simulink model "Simulation_balance_TEST"  (R2024a)
settings: Solver=ode4  StartTime=0.0  StopTime=5  FixedStep=1/750000  RelTol=1e-3
InitFcn:
  | Initialisation_simulation
values from neighbouring files (symbols this model uses):
  denom_com = [R^2*C^2 3*R*C 1]    [Initialisation_simulation.m]
  denom_cou = [1/(2*pi*165) 1]    [Initialisation_simulation.m]
  denom_pos = [1/(2*pi*80) 1]    [Initialisation_simulation.m]
  gain_com = 0.88    [Initialisation_simulation.m]
  gain_cou = 0.716    [Initialisation_simulation.m]
  gain_mod_cou = Gain_Ampli_Puissance(1)    [Initialisation_simulation.m]
  gain_pos = 1.4925    [Initialisation_simulation.m]
  gain_puis = Gain_Ampli_Puissance(1)    [Initialisation_simulation.m]
  num_com = 1    [Initialisation_simulation.m]
  num_cou = 1    [Initialisation_simulation.m]
  num_pos = 1    [Initialisation_simulation.m]
  offset_com = -2.5    [Initialisation_simulation.m]
  offset_cou = 3.44    [Initialisation_simulation.m]
  offset_pos = -1.6    [Initialisation_simulation.m]
  per_adc = 1/freq_adc    (= 0.000166666666667)    [Initialisation_simulation.m]
  per_pwm = 1/freq_pwm    (= 6.4e-05)    [Initialisation_simulation.m]
  sat_com_max = 5    [Initialisation_simulation.m]
  sat_com_min = -5    [Initialisation_simulation.m]
  sat_cou_max = 5    [Initialisation_simulation.m]
  sat_cou_min = 0    [Initialisation_simulation.m]
  sat_pos_max = 5    [Initialisation_simulation.m]
  sat_pos_min = 0    [Initialisation_simulation.m]
  sat_proc_max = 14e-3    (= 0.014)    [Initialisation_simulation.m]    (also in lookup_table_statespace.m = 1)
  sat_proc_min = 0    [Initialisation_simulation.m]    (also in lookup_table_statespace.m = -1)
  sat_puis_max = 5    [Initialisation_simulation.m]
  sat_puis_min = -5    [Initialisation_simulation.m]
  tension_selon_distance = polyfit(Distance(1:point_final), Tension(1:point_final), 3)    [Initialisation_simulation.m]
undefined symbols (not defined in the file or in its folder): denom_pid_cou, denom_pid_pos, denom_proc, num_pid_cou, num_pid_pos, num_proc
libraries: simulink_extras x2, simulink x1
settings Model: DataTypeOverride=Double  MinMaxOverflowLogging=ForceOff  Creator=johen30  LastModifiedBy=johen30

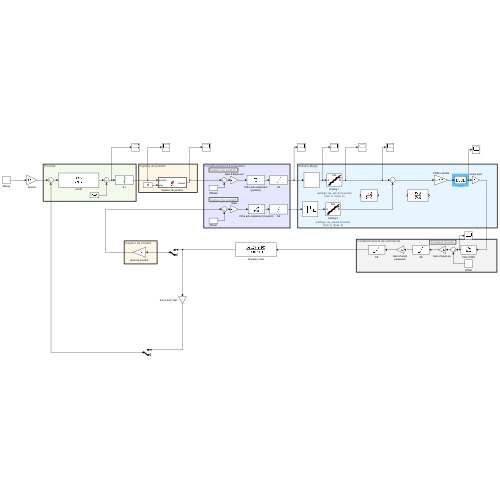
[thumbnail: Simulink's stored preview of the top-level diagram]
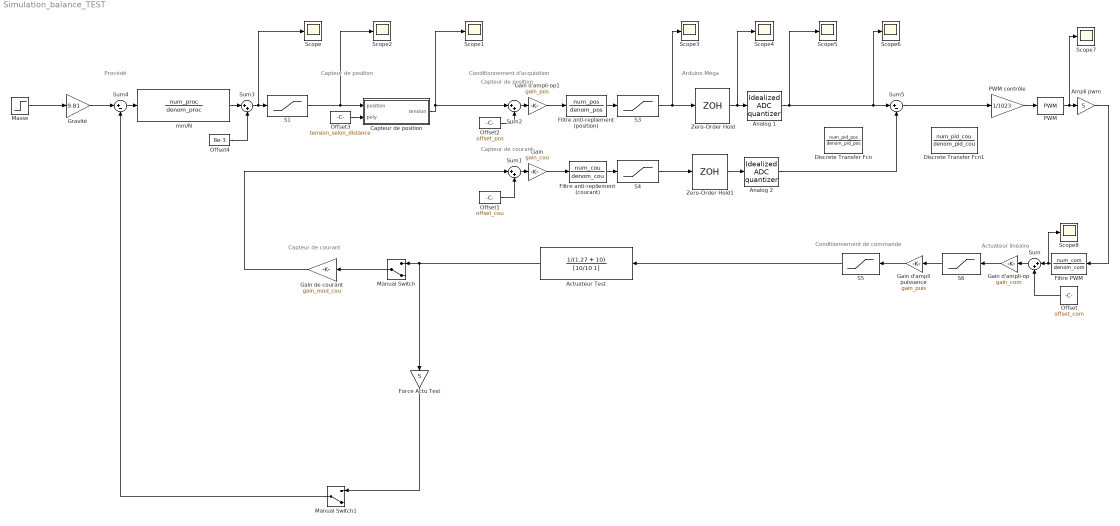
== system Simulation_balance_TEST ==
  note: Conditionnement de commande
  note: Arduino Mega
  note: Capteur de courant
  note: Conditionnement d'acquisition
  note: Procédé
  note: Capteur de position
  note: Actuateur linéaire
  note: Capteur de courant
  note: Capteur de position
  Actuateur Test : TransferFcn  Numerator=1/(1.27 + 10)  Denominator=[10/10 1]
  Ampli pwm : Gain  Gain=5
  Analog 1 : simulink_extras/Additional Discrete/Idealized ADC quantizer  NumberOfConverterBits=res_adc  Vmin=0  Vmax=5  OutputDataType=int16  OutputNegativeValues=off
  Analog 2 : simulink_extras/Additional Discrete/Idealized ADC quantizer  NumberOfConverterBits=res_adc  Vmin=0  Vmax=5  OutputDataType=int16  OutputNegativeValues=off
  Capteur de position : MATLAB Function  TreatAsAtomicUnit=on
  Discrete Transfer Fcn : DiscreteTransferFcn  Numerator=num_pid_pos  Denominator=denom_pid_pos
  Discrete Transfer Fcn1 : DiscreteTransferFcn  Numerator=num_pid_cou  Denominator=denom_pid_cou
  Filtre PWM : TransferFcn  Numerator=num_com  Denominator=denom_com
  Filtre anti-repliement (position) : TransferFcn  Numerator=num_pos  Denominator=denom_pos
  Filtre anti-repliement (courant) : TransferFcn  Numerator=num_cou  Denominator=denom_cou
  Force Actu Test : Gain  Gain=5
  Gain : Gain  Gain=gain_cou
  Gain d'ampli puissance : Gain  Gain=gain_puis
  Gain d'ampli-op : Gain  Gain=gain_com
  Gain d'ampli-op1 : Gain  Gain=gain_pos
  Gain de courant : Gain  Gain=gain_mod_cou
  Gravité : Gain  Gain=9.81
  Manual Switch : ManualSwitch  CurrentSetting=0
  Manual Switch1 : ManualSwitch  CurrentSetting=0
  Masse : Step  After=50e-3  SampleTime=0
  Offset : Constant  Value=offset_com
  Offset1 : Constant  Value=offset_cou
  Offset2 : Constant  Value=offset_pos
  Offset3 : Constant  Value=tension_selon_distance
  Offset4 : Constant  Value=8e-3
  PWM : simulink/Discontinuities/PWM  DisableCoverage=on  Period=per_pwm  InitialDelay=0  DisallowZeroDutyCycle=off  RunAtFixedTimeIntervals=on  SampleTime=1/750000
  PWM contrôle : Gain  Gain=1/1023  OutDataTypeStr=fixdt(1,64, 44)
  S1 : Saturate  UpperLimit=sat_proc_max  LowerLimit=sat_proc_min  LinearizeAsGain=off
  S3 : Saturate  UpperLimit=sat_pos_max  LowerLimit=sat_pos_min  LinearizeAsGain=off
  S4 : Saturate  UpperLimit=sat_cou_max  LowerLimit=sat_cou_min
  S5 : Saturate  UpperLimit=sat_puis_max  LowerLimit=sat_puis_min
  S6 : Saturate  UpperLimit=sat_com_max  LowerLimit=sat_com_min
  Scope{,1..8} (9 alike) : Scope
  Sum{,1..3} (4 alike) : Sum  Inputs=|++
  Sum4 : Sum  Inputs=|+-
  Sum5 : Sum  Inputs=|+-
  Zero-Order Hold : ZeroOrderHold  SampleTime=per_adc
  Zero-Order Hold1 : ZeroOrderHold  SampleTime=per_adc
  mm/N : TransferFcn  Numerator=num_proc  Denominator=denom_proc
  wires:
  Manual Switch/1 -> Gain de courant/1
  Force Actu Test/1 -> Manual Switch1/1
  Sum5/1 -> PWM contrôle/1
  Gain/1 -> Filtre anti-repliement (courant)/1
  Offset2/1 -> Sum2/2
  S1/1 -> Scope2/1, Capteur de position/1(position)
  Zero-Order Hold1/1 -> Analog 2/1
  Sum/1 -> Gain d'ampli-op/1
  S4/1 -> Zero-Order Hold1/1
  Filtre anti-repliement (courant)/1 -> S4/1
  Capteur de position/1(tension) -> Scope1/1, Sum2/1
  PWM/1 -> Scope7/1, Ampli pwm/1
  PWM contrôle/1 -> PWM/1
  S5/1 -> Actuateur Test/1
  Filtre PWM/1 -> Scope8/1, Sum/1
  Gravité/1 -> Sum4/1
  Sum4/1 -> mm/N/1
  Analog 2/1 -> Sum5/2
  S6/1 -> Gain d'ampli puissance/1
  Actuateur Test/1 -> Manual Switch/1, Force Actu Test/1
  S3/1 -> Scope3/1, Zero-Order Hold/1
  Sum2/1 -> Gain d'ampli-op1/1
  Analog 1/1 -> Scope6/1, Sum5/1, Scope5/1
  Offset/1 -> Sum/2
  Ampli pwm/1 -> Filtre PWM/1
  Gain d'ampli-op/1 -> S6/1
  Gain d'ampli puissance/1 -> S5/1
  Zero-Order Hold/1 -> Scope4/1, Analog 1/1
  Filtre anti-repliement (position)/1 -> S3/1
  Gain de courant/1 -> Sum1/1
  Gain d'ampli-op1/1 -> Filtre anti-repliement (position)/1
  Offset1/1 -> Sum1/2
  Sum1/1 -> Gain/1
  Masse/1 -> Gravité/1
  Manual Switch1/1 -> Sum4/2
  Offset3/1 -> Capteur de position/2(poly)
  mm/N/1 -> Sum3/1
  Offset4/1 -> Sum3/2
  Sum3/1 -> Scope/1, S1/1

== matlab function Simulation_balance_TEST/Capteur de position ==
  data: position input; tension output; poly input
function tension = fct(position, poly)

tension = polyval(poly, position);
